simulink model "eeee"  (R2021b)
settings: Solver=VariableStepAuto  StartTime=0.0  StopTime=100  RelTol=1e-3
undefined symbols (not defined in the file): g, l, m, M
settings Model: Creator=vladimirberman  LastModifiedBy=vladimirberman

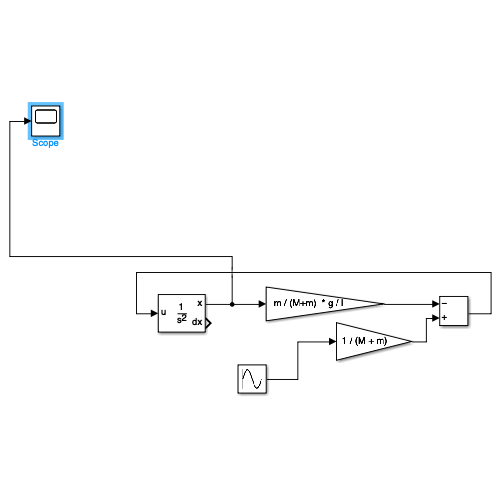
[thumbnail: Simulink's stored preview of the top-level diagram]
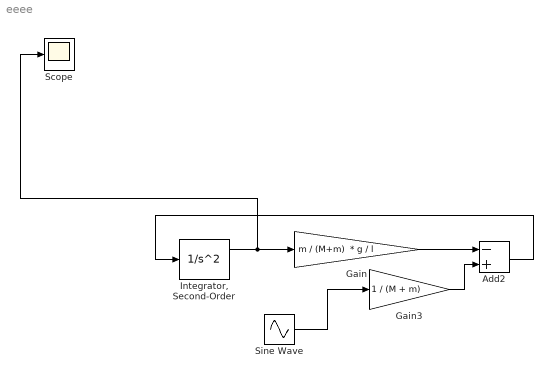
== system eeee ==
  Add2 : Sum  Inputs=-+
  Gain : Gain  Gain="m / (M+m)  * g / l"
  Gain3 : Gain  Gain=1 / (M + m)
  "Integrator, Second-Order" : SecondOrderIntegrator  ICX=0.001
  Scope : Scope
  Sine Wave : Sin  Amplitude=0  SampleTime=0
  wires:
  "Integrator, Second-Order"/1 -> Gain/1, Scope/1
  Gain/1 -> Add2/1
  Gain3/1 -> Add2/2
  Add2/1 -> "Integrator, Second-Order"/1
  Sine Wave/1 -> Gain3/1
